simulink model "ModeloTanquePractica1"  (R2014b)
settings: Solver=ode45  StartTime=0.0  StopTime=10.0  RelTol=1e-3
settings Model: Creator=Andres  LastModifiedBy=Andres

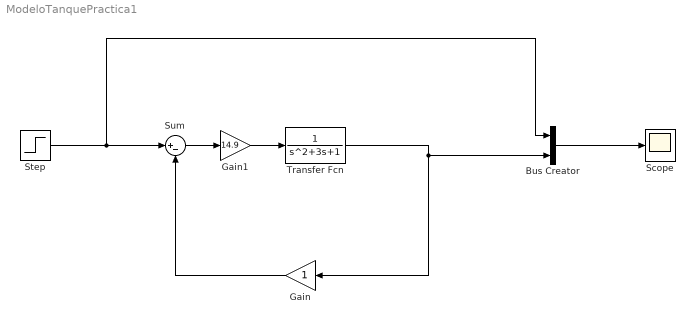
== system ModeloTanquePractica1 ==
  Bus Creator : BusCreator  Inputs=2
  Gain : Gain
  Gain1 : Gain  Gain=14.9
  Scope : Scope
  Step : Step  Time=0  SampleTime=0
  Sum : Sum  Inputs=|+-
  Transfer Fcn : TransferFcn  Denominator=[1 3 1]
  wires:
  Transfer Fcn/1 -> Bus Creator/2, Gain/1
  Gain/1 -> Sum/2
  Bus Creator/1 -> Scope/1
  Step/1 -> Bus Creator/1, Sum/1
  Sum/1 -> Gain1/1
  Gain1/1 -> Transfer Fcn/1
